simulink model "model_sinMR_MdE"  (R2021b)
settings: Solver=ode4  StartTime=0.0  StopTime=tend  FixedStep=ts  RelTol=1e-3  EnableMultiTasking=on
values from neighbouring files (symbols this model uses):
  ct = 2*mt*(2*pi*ft)*dampt    [Run_MdE_Research_Report.m]    (also in my_script.m)
  Kmax = 50*ct    [Run_MdE_Research_Report.m]    (also in my_script.m)
  Kmin = ct/2    [Run_MdE_Research_Report.m]    (also in my_script.m)
  kt = ((2*pi*ft)^2)*mt    [Run_MdE_Research_Report.m]    (also in Run_MdE_Research_Report_con_MR_damper.m; my_script.m)
  mt = mu*m1    (= 0.02)    [Run_MdE_Research_Report.m]    (also in Run_MdE_Research_Report_con_MR_damper.m = 40; my_script.m)
  tend = 500    [Run_MdE_Research_Report.m]    (also in Run_MdE_Research_Report_con_MR_damper.m; my_script.m)
  ts = 1/fs    (= 0.000666666666667)    [Run_MdE_Research_Report.m]    (also in Run_MdE_Research_Report_con_MR_damper.m; my_script.m)
undefined symbols (not defined in the file or in its folder): D_Gs, N_Gs
libraries: simulink x1
settings Model: Creator=user  LastModifiedBy=Jose Manuel Soria
settings SolverCC: AlgebraicLoopSolver=TrustRegion
settings DataIOCC: LimitDataPoints=on  SaveFormat=Array  SignalLoggingSaveFormat=ModelDataLogs  ReturnWorkspaceOutputs=off  SignalLoggingName=sigsOut
settings OptimizationCC: InitFltsAndDblsToZero=on  LifeSpan=inf
settings DebuggingCC: SaveWithParameterizedLinksMsg=none  UnderspecifiedInitializationDetection=Classic  MergeDetectMultiDrivingBlocksExec=none  SignalResolutionControl=TryResolveAllWithWarning  MultiTaskDSMMsg=warning  MultiTaskCondExecSysMsg=none  FcnCallInpInsideContextMsg=warning  SFUnexpectedBacktrackingDiag=warning  SFNoUnconditionalDefaultTransitionDiag=warning  SFMachineParentedDataDiag=warning  ArithmeticOperatorsInVariantConditions=warning
settings HardwareCC: ProdBitPerPointer=32  ProdBitPerSizeT=32  ProdBitPerPtrDiffT=32  ProdLargestAtomicFloat=None  ProdIntDivRoundTo=Undefined  ProdEndianess=Unspecified  ProdWordSize=32  ProdHWDeviceType=32-bit Generic  TargetBitPerPointer=64  TargetBitPerSizeT=64  TargetBitPerPtrDiffT=64  TargetLongLongMode=on  TargetIntDivRoundTo=Zero  TargetEndianess=LittleEndian  TargetWordSize=64  TargetHWDeviceType=MATLAB Host  ProdEqTarget=off
settings ModelReferenceCC: PropagateSignalLabelsOutOfModel=off
settings SFSimCC: SimUseLocalCustomCode=off  CustomCodeUndefinedFunction=UseInterfaceOnly
settings RTWCC: RTWUseLocalCustomCode=off
settings CodeAppCC: StateflowObjectComments=on
settings GRTTargetCC: TargetFcnLib=ansi_tfl_tmw.mat  TargetLangStandard=C89/C90 (ANSI)  CombineOutputUpdateFcns=off  GRTInterface=on
settings ConfigComp: CovMetricSettings=dw  CovSaveCumulativeToWorkspaceVar=on  CovSaveSingleToWorkspaceVar=on  CovExternalEMLEnable=off  CovSFcnEnable=off

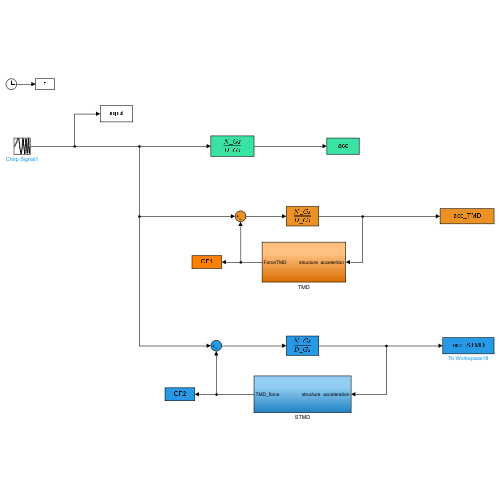
[thumbnail: Simulink's stored preview of the top-level diagram]
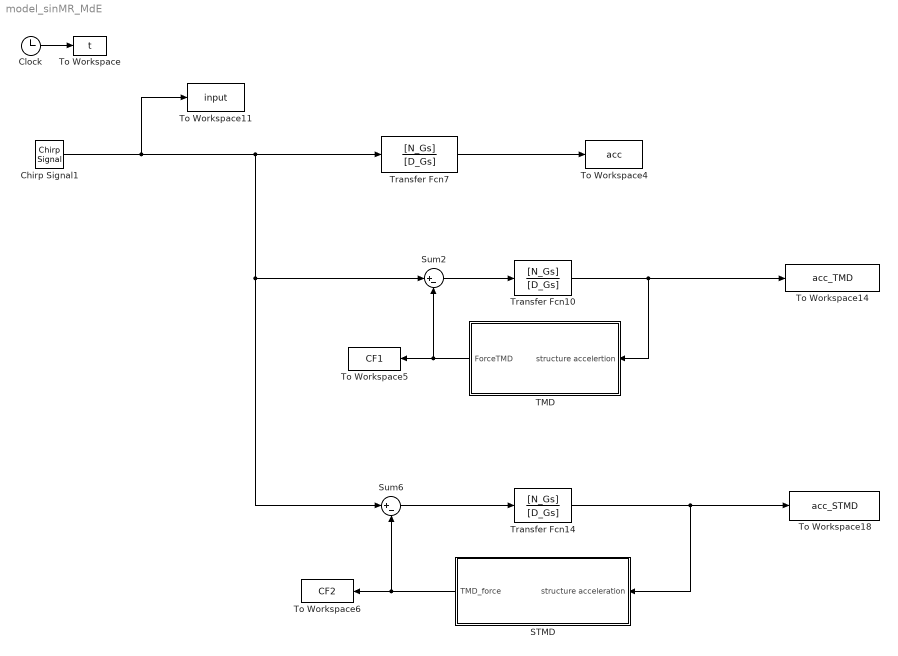
== system model_sinMR_MdE ==
  Chirp Signal1 : simulink/Sources/Chirp Signal  f1=fmin  T=tend  f2=fmax
  Clock : Clock
  STMD : Subsystem
  Sum2 : Sum  Inputs=|+-
  Sum6 : Sum  Inputs=|+-
  TMD : Subsystem
  To Workspace : ToWorkspace  VariableName=t  SampleTime=ts
  To Workspace11 : ToWorkspace  VariableName=input  SampleTime=ts
  To Workspace14 : ToWorkspace  VariableName=acc_TMD  SampleTime=ts
  To Workspace18 : ToWorkspace  VariableName=acc_STMD  SampleTime=ts
  To Workspace4 : ToWorkspace  VariableName=acc  SampleTime=ts
  To Workspace5 : ToWorkspace  VariableName=CF1  SampleTime=ts
  To Workspace6 : ToWorkspace  VariableName=CF2  SampleTime=ts
  Transfer Fcn10 : TransferFcn  Numerator=[N_Gs]  Denominator=[D_Gs]
  Transfer Fcn14 : TransferFcn  Numerator=[N_Gs]  Denominator=[D_Gs]
  Transfer Fcn7 : TransferFcn  Numerator=[N_Gs]  Denominator=[D_Gs]
  wires:
  Clock/1 -> To Workspace/1
  Sum2/1 -> Transfer Fcn10/1
  TMD/1(ForceTMD) -> Sum2/2, To Workspace5/1
  Transfer Fcn7/1 -> To Workspace4/1
  Transfer Fcn10/1 -> TMD/1(structure accelertion), To Workspace14/1
  Sum6/1 -> Transfer Fcn14/1
  Transfer Fcn14/1 -> STMD/1(structure acceleration), To Workspace18/1
  STMD/1(TMD_force) -> Sum6/2, To Workspace6/1
  Chirp Signal1/1 -> Transfer Fcn7/1, Sum2/1, Sum6/1, To Workspace11/1

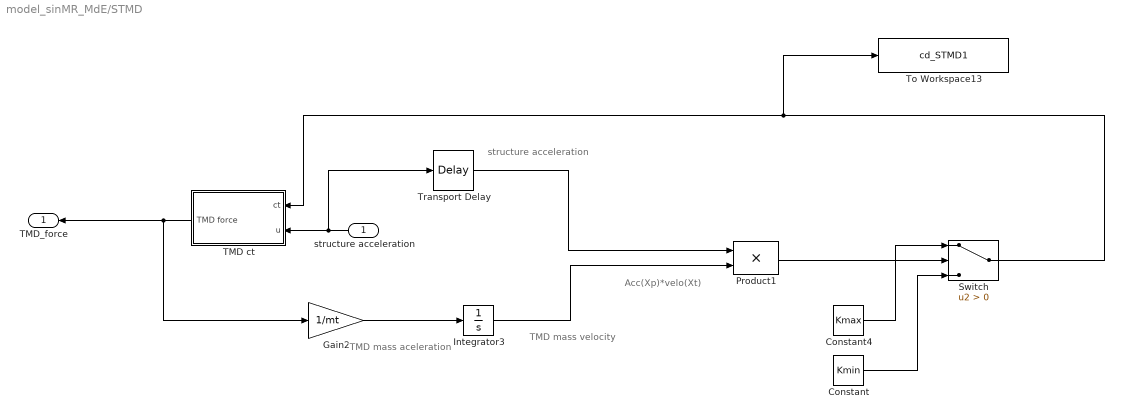
== system model_sinMR_MdE/STMD ==
  note: structure acceleration
  note: TMD mass
      | aceleration
  note: Acc(Xp)*velo(Xt)
  note: TMD mass
      | velocity
  structure acceleration : Inport
  Constant : Constant  Value=Kmin
  Constant4 : Constant  Value=Kmax
  Gain2 : Gain  Gain=1/mt
  Integrator3 : Integrator
  Product1 : Product  OutDataTypeStr=double  SaturateOnIntegerOverflow=on
  Switch : Switch  Criteria=u2 > Threshold
  TMD ct : Subsystem
  To Workspace13 : ToWorkspace  VariableName=cd_STMD1  SampleTime=ts
  Transport Delay : TransportDelay  DelayTime=ts
  TMD_force : Outport  VectorParamsAs1DForOutWhenUnconnected=off
  wires:
  TMD ct/1(TMD force) -> Gain2/1, TMD_force/1
  Integrator3/1 -> Product1/2
  Switch/1 -> To Workspace13/1, TMD ct/1(ct)
  structure acceleration/1 -> Transport Delay/1, TMD ct/2(u)
  Transport Delay/1 -> Product1/1
  Gain2/1 -> Integrator3/1
  Product1/1 -> Switch/2
  Constant4/1 -> Switch/1
  Constant/1 -> Switch/3

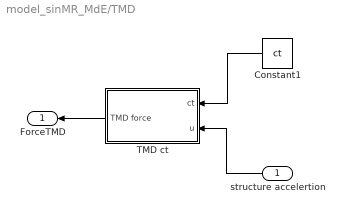
== system model_sinMR_MdE/TMD ==
  structure accelertion : Inport
  Constant1 : Constant  Value=ct
  TMD ct : Subsystem
  ForceTMD : Outport  VectorParamsAs1DForOutWhenUnconnected=off
  wires:
  TMD ct/1(TMD force) -> ForceTMD/1
  structure accelertion/1 -> TMD ct/2(u)
  Constant1/1 -> TMD ct/1(ct)

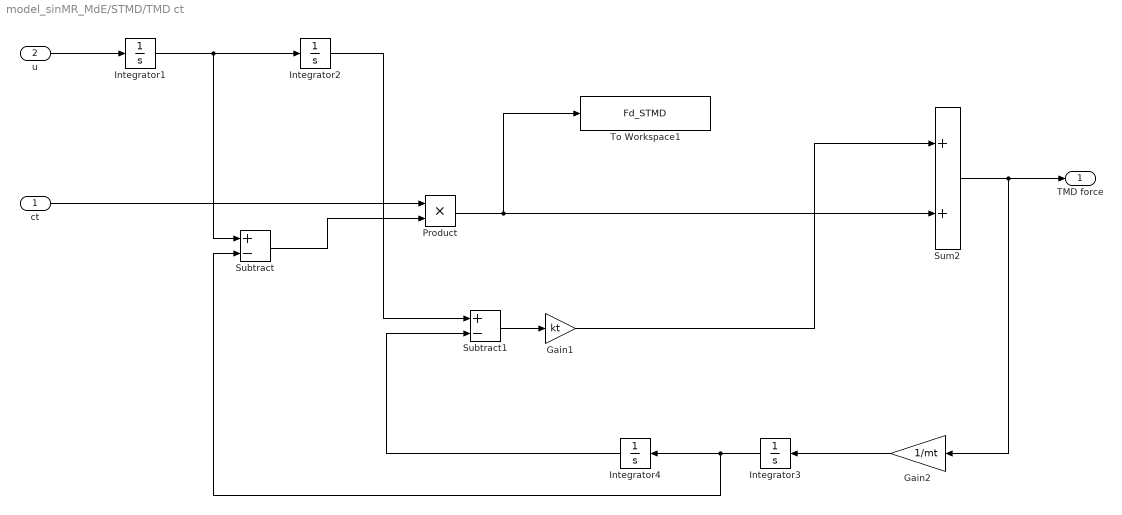
== system model_sinMR_MdE/STMD/TMD ct ==
  ct : Inport
  u : Inport  Port=2
  Gain1 : Gain  Gain=kt
  Gain2 : Gain  Gain=1/mt
  Integrator{1..4} (4 alike) : Integrator
  Product : Product
  Subtract : Sum  Inputs=+-
  Subtract1 : Sum  Inputs=+-
  Sum2 : Sum
  To Workspace1 : ToWorkspace  VariableName=Fd_STMD  SampleTime=ts
  TMD force : Outport  VectorParamsAs1DForOutWhenUnconnected=off
  wires:
  Integrator1/1 -> Subtract/1, Integrator2/1
  u/1 -> Integrator1/1
  Integrator3/1 -> Integrator4/1, Subtract/2
  Gain2/1 -> Integrator3/1
  Integrator4/1 -> Subtract1/2
  Integrator2/1 -> Subtract1/1
  Subtract1/1 -> Gain1/1
  Gain1/1 -> Sum2/1
  Sum2/1 -> Gain2/1, TMD force/1
  ct/1 -> Product/1
  Subtract/1 -> Product/2
  Product/1 -> Sum2/2, To Workspace1/1

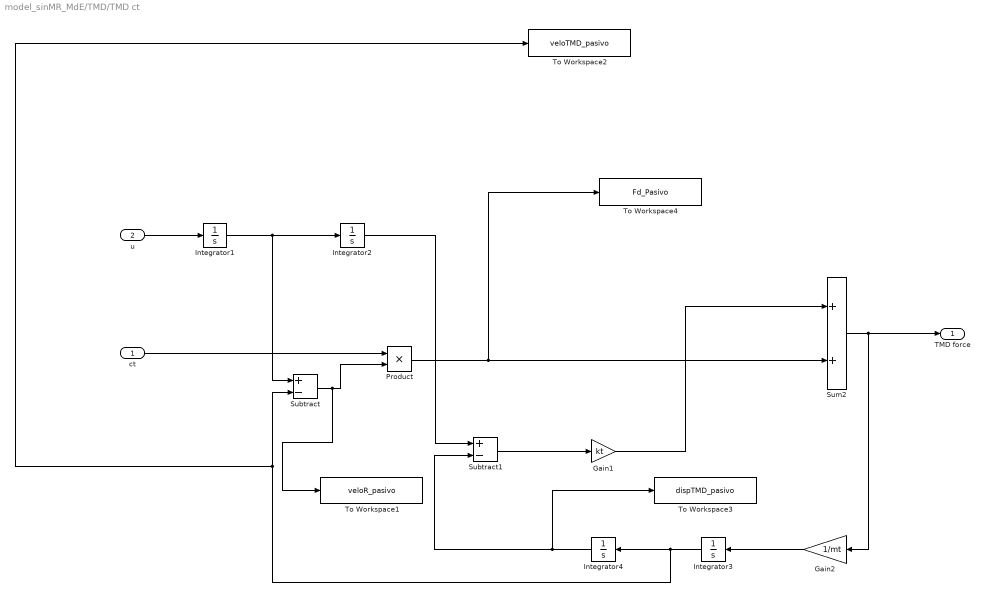
== system model_sinMR_MdE/TMD/TMD ct ==
  ct : Inport
  u : Inport  Port=2
  Gain1 : Gain  Gain=kt
  Gain2 : Gain  Gain=1/mt
  Integrator{1..4} (4 alike) : Integrator
  Product : Product
  Subtract : Sum  Inputs=+-
  Subtract1 : Sum  Inputs=+-
  Sum2 : Sum
  To Workspace1 : ToWorkspace  VariableName=veloR_pasivo  SampleTime=ts
  To Workspace2 : ToWorkspace  VariableName=veloTMD_pasivo  SampleTime=ts
  To Workspace3 : ToWorkspace  VariableName=dispTMD_pasivo  SampleTime=ts
  To Workspace4 : ToWorkspace  VariableName=Fd_Pasivo  SampleTime=ts
  TMD force : Outport  VectorParamsAs1DForOutWhenUnconnected=off
  wires:
  Integrator1/1 -> Subtract/1, Integrator2/1
  u/1 -> Integrator1/1
  ct/1 -> Product/1
  Integrator3/1 -> Integrator4/1, To Workspace2/1, Subtract/2
  Subtract/1 -> To Workspace1/1, Product/2
  Gain2/1 -> Integrator3/1
  Integrator4/1 -> To Workspace3/1, Subtract1/2
  Integrator2/1 -> Subtract1/1
  Subtract1/1 -> Gain1/1
  Gain1/1 -> Sum2/1
  Sum2/1 -> Gain2/1, TMD force/1
  Product/1 -> Sum2/2, To Workspace4/1
